simulink model "motor_torque_inverter"  (R2022b)
settings: Solver=ode23t  StartTime=0.0  StopTime=0.1  MaxStep=1e-6  RelTol=1e-6  AbsTol=1e-6
undefined symbols (not defined in the file): Jeq, K, Ki_cc, Kp_cc, La, Ra
libraries: spsMosfetLib x4, spsCurrentMeasurementLib x1, spsDCMachineLib x1, spsDCVoltageSourceLib x1, simulink x1, spspowerguiLib x1
settings Model: Creator=NT550XDA-KC35W  LastModifiedBy=NT550XDA-KC35W

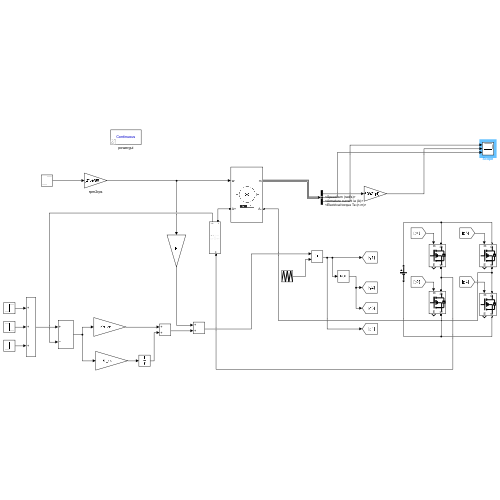
[thumbnail: Simulink's stored preview of the top-level diagram]
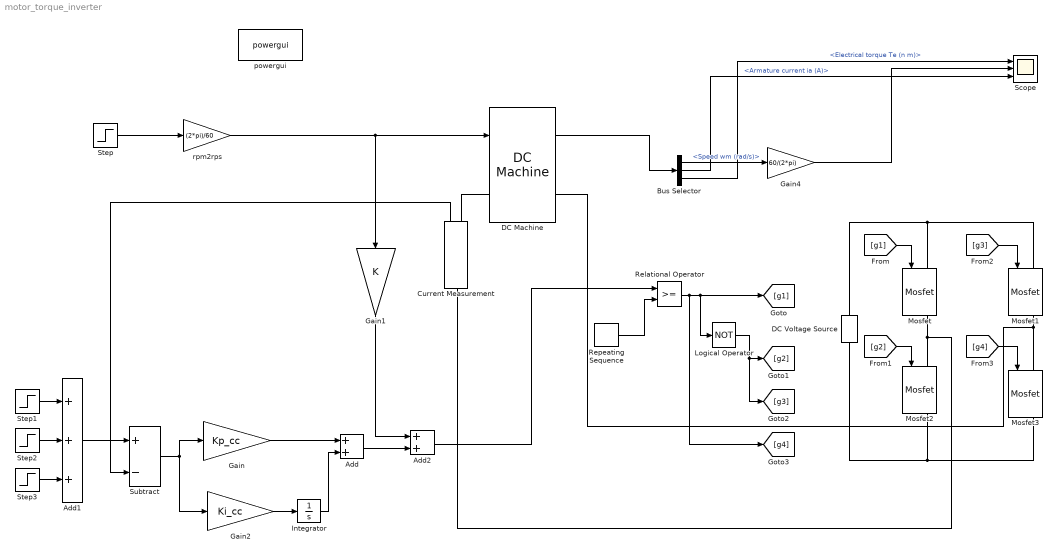
== system motor_torque_inverter ==
  Add : Sum
  Add1 : Sum  Inputs=+++
  Add2 : Sum
  Bus Selector : BusSelector  OutputSignals=Speed wm (rad/s),Armature current ia (A),Electrical torque Te (n m)
  Current Measurement : spsCurrentMeasurementLib/Current Measurement  PhasorSimulation=off  OutputType=Complex  PSBequivalent=0
  DC Machine : spsDCMachineLib/DC Machine  PresetModel=No  MechanicalLoad=Speed w  FieldType=Permanent magnet  ShowDetailedParameters=on  MeasurementBus=off  RLa="[ Ra  La]"  RLf="[ 240  120]"  Laf=1.8  MachineConstant=Back-emf constant (V/rpm)  Ke=K*2*pi/60  Kt=1.8  J=Jeq  Bm=Beq  Tf=0  w0=0  Ifinit=1  TsPowergui=0  TsBlock=-1
  DC Voltage Source : spsDCVoltageSourceLib/DC Voltage Source  Amplitude=120  Measurements=None
  Gain : Gain  Gain=Kp_cc
  Gain1 : Gain  Gain=K
  Gain2 : Gain  Gain=Ki_cc
  Gain4 : Gain  Gain=60/(2*pi)
  Integrator : Integrator
  Logical Operator : Logic  Operator=NOT  AllPortsSameDT=off  OutDataTypeStr=boolean
  Mosfet{,1..3} (4 alike) : spsMosfetLib/Mosfet  Ron=0.1  Lon=0  Rd=0.01  Vfd=0  IC=0  Rs=1e5  Cs=inf  Measurements=on
  Relational Operator : RelationalOperator  OutDataTypeStr=boolean  RndMeth=Simplest  InputSameDT=off
  Repeating Sequence : simulink/Sources/Repeating Sequence  rep_seq_t=[0 0.00005 0.0001]  rep_seq_y=[-120 120 -120]
  Scope : Scope  NumInputPorts=3
  Step : Step  Time=0.02  After=1300  SampleTime=0
  Step1 : Step  Time=0.01  After=15  SampleTime=0
  Step2 : Step  Time=0.06  After=-15  SampleTime=0
  Step3 : Step  Time=0.08  After=15  SampleTime=0
  Subtract : Sum  Inputs=+-
  powergui : spspowerguiLib/powergui  Priority=1  SimulationMode=Continuous  SampleTime=50e-6  frequency=60  Iterations=50  frequencyindice=0  Pbase=100e6  ErrMax=1e-4  UnitsV=kV  UnitsW=MW  buscounter=0  FunctionMessages=off  echomessages=off  EnableUseOfTLC=off  CurrentSourceSwitches=off  DisableSnubberDevices=off  DisableRonSwitches=off  DisableVfSwitches=off  DisplayEquations=off  AutomaticDiscreteSolvers=off  SolverType=Tustin/Backward Euler (TBE)  Interpol=off  ExternalGateDelay=off  methode=off  Ts=100  x0status=blocks  SPID=on  SwTol=0  HookPort=off  NonlinearTolerance=1e-4  nMaxIteration=100  ContinueOnMaxIteration=off  RestoreLinks=warning  ResistiveCurrentMeasurement=off  Frange=[0:2:500]  Ylog=off  Xlog=on  ShowGrid=off  save=off  variable=ZData  structure=0  ZoomFFT=off  StartTime=0.0  cycles=1  DisplayStyle=1  fundamental=60  FreqAxis=off  MaxFrequency=1000  frequencyindicesteady=1  RmsSteady=1  display=off
  rpm2rps : Gain  Gain=(2*pi)/60
  wires:
  DC Machine/1 -> Bus Selector/1
  Bus Selector/1 -> Gain4/1  "<Speed wm (rad/s)>"
  Gain4/1 -> Scope/2
  Bus Selector/2 -> Scope/3  "<Armature current ia (A)>"
  Bus Selector/3 -> Scope/1  "<Electrical torque Te (n m)>"
  Gain2/1 -> Integrator/1
  Gain/1 -> Add/1
  Integrator/1 -> Add/2
  Subtract/1 -> Gain/1, Gain2/1
  Add/1 -> Add2/2
  Current Measurement/1 -> Subtract/2
  rpm2rps/1 -> Gain1/1, DC Machine/1
  Step/1 -> rpm2rps/1
  Add1/1 -> Subtract/1
  Step1/1 -> Add1/1
  Step2/1 -> Add1/2
  Step3/1 -> Add1/3
  Gain1/1 -> Add2/1
  [g1] -> Mosfet/1
  [g2] -> Mosfet2/1
  [g3] -> Mosfet1/1
  [g4] -> Mosfet3/1
  Repeating Sequence/1 -> Relational Operator/2
  Relational Operator/1 -> [g4], Logical Operator/1, [g1]
  Logical Operator/1 -> [g3], [g2]
  Add2/1 -> Relational Operator/1
  connections:
  Mosfet1/RConn1 -- DC Machine/RConn1 -- Mosfet3/LConn1
  Current Measurement/RConn1 -- DC Machine/LConn1
  Mosfet3/RConn1 -- DC Voltage Source/LConn1 -- Mosfet2/RConn1
  DC Voltage Source/RConn1 -- Mosfet/LConn1 -- Mosfet1/LConn1
  Mosfet/RConn1 -- Current Measurement/LConn1 -- Mosfet2/LConn1
